simulink subsystem "GasToAlpha"  (R2021b)
settings: Solver=VariableStepAuto  StartTime=0.0  StopTime=10.0  RelTol=1e-3
settings Model: Creator=silen  LastModifiedBy=Jiaqi

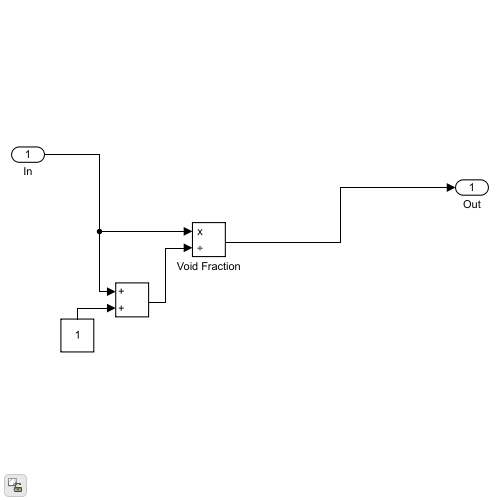
[thumbnail: Simulink's stored preview of the top-level diagram]
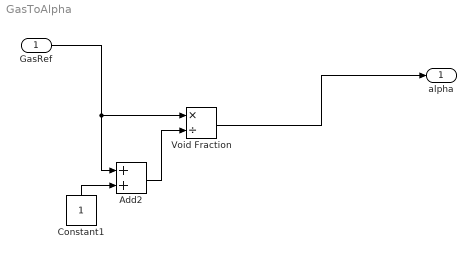
== system GasToAlpha ==
  GasRef : Inport
  Add2 : Sum
  Constant1 : Constant
  Void Fraction : Product  Inputs=*/
  alpha : Outport
  wires:
  Add2/1 -> Void Fraction/2
  Constant1/1 -> Add2/2
  Void Fraction/1 -> alpha/1
  GasRef/1 -> Add2/1, Void Fraction/1
